simulink model "Aufg7_1"  (R2018a)
settings: Solver=VariableStepDiscrete  StartTime=0.0  StopTime=60  MaxStep=inf  RelTol=1e-3
undefined symbols (not defined in the file or in its folder): des, gcbh
settings Model: Creator=Naveen  LastModifiedBy=Naveen
settings DataIOCC: ReturnWorkspaceOutputs=on
settings SFSimCC: SimUseLocalCustomCode=on
settings RTWCC: RTWUseLocalCustomCode=on

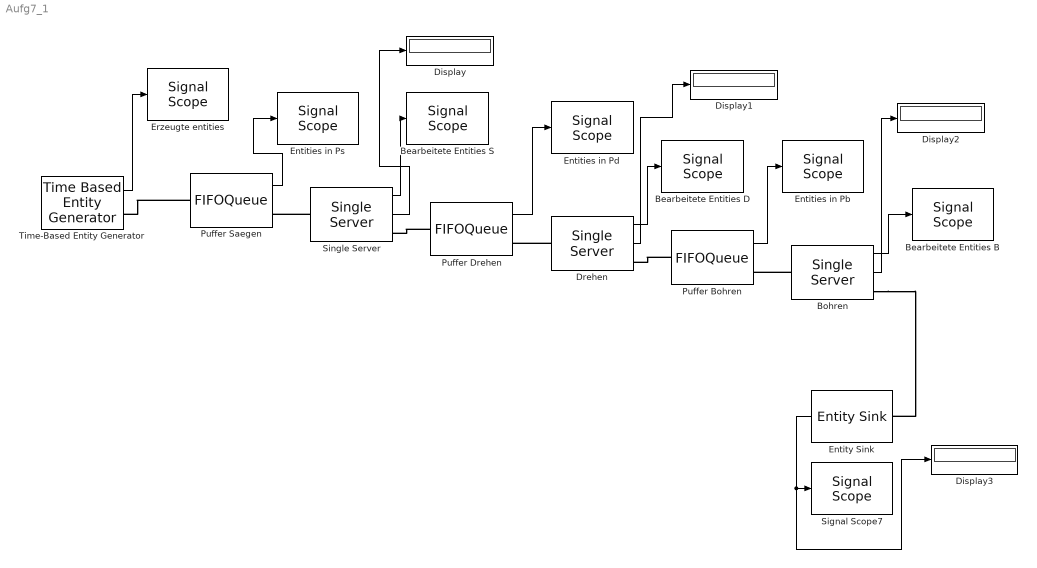
== system Aufg7_1 ==
  Bearbeitete Entities B : SignalScope  LoadFcn=des.scope.CallbackSupport('seLoadFcn',gcbh)  StartFcn=des.scope.CallbackSupport('seStartFcn',gcbh)  StopFcn=des.scope.CallbackSupport('seStopFcn',gcbh)
      settings: CopyFcn=des.scope.CallbackSupport('seCopyFcn',gcbh)  DeleteFcn=des.scope.CallbackSupport('seDeleteFcn',gcbh)  PreSaveFcn=des.scope.CallbackSupport('sePreSaveFcn',gcbh)  NameChangeFcn=des.scope.CallbackSupport('seNameChangeFcn',gcbh)  OpenFcn=des.scope.CallbackSupport('seOpenFcn',gcbh)
  Bearbeitete Entities D : SignalScope  LoadFcn=des.scope.CallbackSupport('seLoadFcn',gcbh)  StartFcn=des.scope.CallbackSupport('seStartFcn',gcbh)  StopFcn=des.scope.CallbackSupport('seStopFcn',gcbh)
      settings: CopyFcn=des.scope.CallbackSupport('seCopyFcn',gcbh)  DeleteFcn=des.scope.CallbackSupport('seDeleteFcn',gcbh)  PreSaveFcn=des.scope.CallbackSupport('sePreSaveFcn',gcbh)  NameChangeFcn=des.scope.CallbackSupport('seNameChangeFcn',gcbh)  OpenFcn=des.scope.CallbackSupport('seOpenFcn',gcbh)
  Bearbeitete Entities S : SignalScope  LoadFcn=des.scope.CallbackSupport('seLoadFcn',gcbh)  StartFcn=des.scope.CallbackSupport('seStartFcn',gcbh)  StopFcn=des.scope.CallbackSupport('seStopFcn',gcbh)
      settings: CopyFcn=des.scope.CallbackSupport('seCopyFcn',gcbh)  DeleteFcn=des.scope.CallbackSupport('seDeleteFcn',gcbh)  PreSaveFcn=des.scope.CallbackSupport('sePreSaveFcn',gcbh)  NameChangeFcn=des.scope.CallbackSupport('seNameChangeFcn',gcbh)  OpenFcn=des.scope.CallbackSupport('seOpenFcn',gcbh)
  Bohren : SingleServer  ServiceTime=ts_bohr  StatNumberDeparted=on  StatUtilization=on
      settings: OutputPortMap=o0,o5
  Display{,1..3} (4 alike) : Display
  Drehen : SingleServer  ServiceTime=ts_dreh  StatNumberDeparted=on  StatUtilization=on
      settings: OutputPortMap=o0,o5
  Entities in Pb : SignalScope  LoadFcn=des.scope.CallbackSupport('seLoadFcn',gcbh)  StartFcn=des.scope.CallbackSupport('seStartFcn',gcbh)  StopFcn=des.scope.CallbackSupport('seStopFcn',gcbh)
      settings: CopyFcn=des.scope.CallbackSupport('seCopyFcn',gcbh)  DeleteFcn=des.scope.CallbackSupport('seDeleteFcn',gcbh)  PreSaveFcn=des.scope.CallbackSupport('sePreSaveFcn',gcbh)  NameChangeFcn=des.scope.CallbackSupport('seNameChangeFcn',gcbh)  OpenFcn=des.scope.CallbackSupport('seOpenFcn',gcbh)
  Entities in Pd : SignalScope  LoadFcn=des.scope.CallbackSupport('seLoadFcn',gcbh)  StartFcn=des.scope.CallbackSupport('seStartFcn',gcbh)  StopFcn=des.scope.CallbackSupport('seStopFcn',gcbh)
      settings: CopyFcn=des.scope.CallbackSupport('seCopyFcn',gcbh)  DeleteFcn=des.scope.CallbackSupport('seDeleteFcn',gcbh)  PreSaveFcn=des.scope.CallbackSupport('sePreSaveFcn',gcbh)  NameChangeFcn=des.scope.CallbackSupport('seNameChangeFcn',gcbh)  OpenFcn=des.scope.CallbackSupport('seOpenFcn',gcbh)
  Entities in Ps : SignalScope  LoadFcn=des.scope.CallbackSupport('seLoadFcn',gcbh)  StartFcn=des.scope.CallbackSupport('seStartFcn',gcbh)  StopFcn=des.scope.CallbackSupport('seStopFcn',gcbh)
      settings: CopyFcn=des.scope.CallbackSupport('seCopyFcn',gcbh)  DeleteFcn=des.scope.CallbackSupport('seDeleteFcn',gcbh)  PreSaveFcn=des.scope.CallbackSupport('sePreSaveFcn',gcbh)  NameChangeFcn=des.scope.CallbackSupport('seNameChangeFcn',gcbh)  OpenFcn=des.scope.CallbackSupport('seOpenFcn',gcbh)
  Entity Sink : EntitySink  StatNumberArrived=on
  Erzeugte entities : SignalScope  LoadFcn=des.scope.CallbackSupport('seLoadFcn',gcbh)  StartFcn=des.scope.CallbackSupport('seStartFcn',gcbh)  StopFcn=des.scope.CallbackSupport('seStopFcn',gcbh)
      settings: CopyFcn=des.scope.CallbackSupport('seCopyFcn',gcbh)  DeleteFcn=des.scope.CallbackSupport('seDeleteFcn',gcbh)  PreSaveFcn=des.scope.CallbackSupport('sePreSaveFcn',gcbh)  NameChangeFcn=des.scope.CallbackSupport('seNameChangeFcn',gcbh)  OpenFcn=des.scope.CallbackSupport('seOpenFcn',gcbh)
  Puffer Bohren : FIFOQueue  Capacity=inf  StatNumberInBlock=on
      settings: OutputPortMap=o1
  Puffer Drehen : FIFOQueue  Capacity=10  StatNumberInBlock=on
      settings: OutputPortMap=o1
  Puffer Saegen : FIFOQueue  Capacity=inf  StatNumberInBlock=on
      settings: OutputPortMap=o1
  Signal Scope7 : SignalScope  LoadFcn=des.scope.CallbackSupport('seLoadFcn',gcbh)  StartFcn=des.scope.CallbackSupport('seStartFcn',gcbh)  StopFcn=des.scope.CallbackSupport('seStopFcn',gcbh)
      settings: CopyFcn=des.scope.CallbackSupport('seCopyFcn',gcbh)  DeleteFcn=des.scope.CallbackSupport('seDeleteFcn',gcbh)  PreSaveFcn=des.scope.CallbackSupport('sePreSaveFcn',gcbh)  NameChangeFcn=des.scope.CallbackSupport('seNameChangeFcn',gcbh)  OpenFcn=des.scope.CallbackSupport('seOpenFcn',gcbh)
  Single Server : SingleServer  ServiceTime=ts_sage  StatNumberDeparted=on  StatUtilization=on
      settings: OutputPortMap=o0,o5
  Time-Based Entity Generator : TimeBasedEntityGenerator  StatNumberDeparted=on
  wires:
  Puffer Saegen/1 -> Entities in Ps/1
  Single Server/1 -> Bearbeitete Entities S/1
  Puffer Drehen/1 -> Entities in Pd/1
  Drehen/1 -> Bearbeitete Entities D/1
  Puffer Bohren/1 -> Entities in Pb/1
  Bohren/1 -> Bearbeitete Entities B/1
  Time-Based Entity Generator/1 -> Erzeugte entities/1
  Entity Sink/1 -> Display3/1, Signal Scope7/1
  Single Server/2 -> Display/1
  Bohren/2 -> Display2/1
  Drehen/2 -> Display1/1
  connections:
  Puffer Saegen/LConn1 -- Time-Based Entity Generator/RConn1
  Single Server/LConn1 -- Puffer Saegen/RConn1
  Puffer Drehen/LConn1 -- Single Server/RConn1
  Drehen/LConn1 -- Puffer Drehen/RConn1
  Puffer Bohren/LConn1 -- Drehen/RConn1
  Bohren/LConn1 -- Puffer Bohren/RConn1
  Bohren/RConn1 -- Entity Sink/LConn1
